simulink model "threee_way"  (R2025b)
settings: Solver=VariableStepAuto  StartTime=0.0  StopTime=0.002  RelTol=1e-3
undefined symbols (not defined in the file or in its folder): dspblkCoreblockFVToolHelper, gcbh
libraries: simulink x4
settings Model: Creator=janek  LastModifiedBy=janek

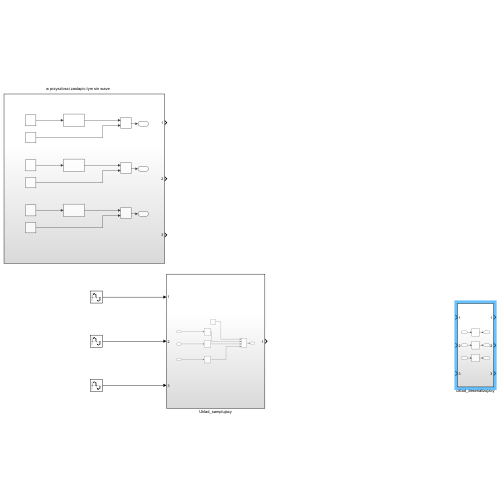
[thumbnail: Simulink's stored preview of the top-level diagram]
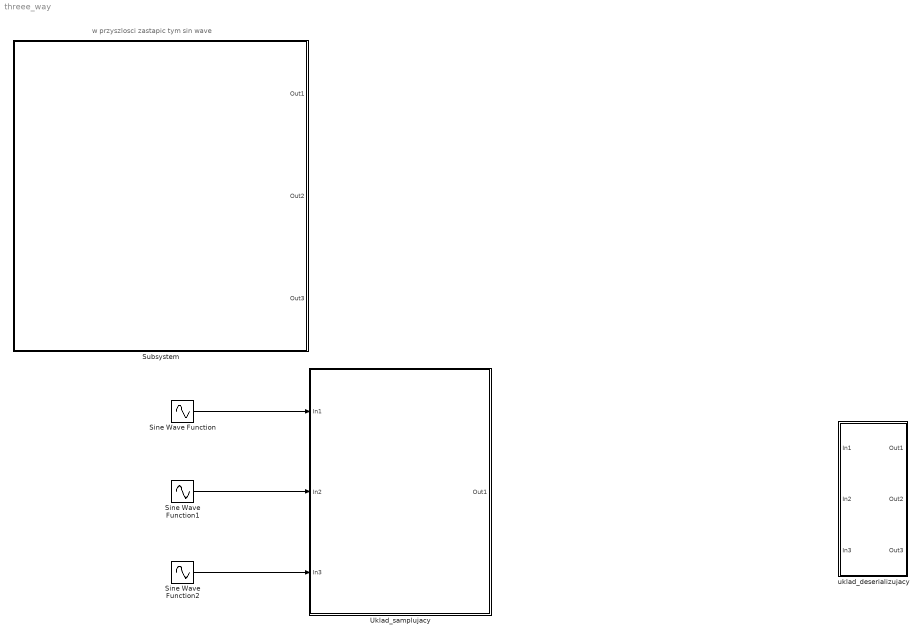
== system threee_way ==
  note: w przyszlosci zastapic tym sin wave
  Sine Wave Function : Sin  Frequency=2*pi*4000  SampleTime=1/27000
  Sine Wave Function1 : Sin  Frequency=2*pi*5000  SampleTime=1/27000
  Sine Wave Function2 : Sin  Frequency=2*pi*3000  SampleTime=1/27000
  Subsystem : Subsystem
  Uklad_samplujacy : Subsystem
  uklad_deserializujacy : Subsystem
  wires:
  Sine Wave Function/1 -> Uklad_samplujacy/1(In1)
  Sine Wave Function1/1 -> Uklad_samplujacy/2(In2)
  Sine Wave Function2/1 -> Uklad_samplujacy/3(In3)

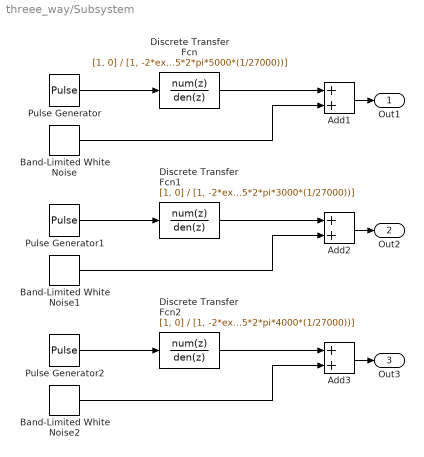
== system threee_way/Subsystem ==
  Add1 : Sum
  Add2 : Sum
  Add3 : Sum
  Band-Limited White Noise : simulink/Sources/Band-Limited White Noise  Cov=[0.000005]  Ts=1/27000  seed=[23341]
  Band-Limited White Noise1 : simulink/Sources/Band-Limited White Noise  Cov=[0.000005]  Ts=1/27000  seed=[23341]
  Band-Limited White Noise2 : simulink/Sources/Band-Limited White Noise  Cov=[0.000005]  Ts=1/27000  seed=[23341]
  Discrete Transfer Fcn : DiscreteTransferFcn  LoadFcn=dspblkCoreblockFVToolHelper(gcbh,'load');  Numerator=[1, 0]  Denominator=[1, -2*exp(-0.05*2*pi*5000*(1/27000))*cos(2*pi*5000*sqrt(1-0.05^2)*(1/27000)), exp(-2*0.05*2*pi*5000*(1/27000))]
      settings: CopyFcn=dspblkCoreblockFVToolHelper(gcbh,'copy');  DeleteFcn=dspblkCoreblockFVToolHelper(gcbh,'close');  ModelCloseFcn=dspblkCoreblockFVToolHelper(gcbh,'close');  PreSaveFcn=dspblkCoreblockFVToolHelper(gcbh,'presave');  PostSaveFcn=dspblkCoreblockFVToolHelper(gcbh,'postsave');  CloseFcn=dspblkCoreblockFVToolHelper(gcbh,'close');
  Discrete Transfer Fcn1 : DiscreteTransferFcn  LoadFcn=dspblkCoreblockFVToolHelper(gcbh,'load');  Numerator=[1, 0]  Denominator=[1, -2*exp(-0.05*2*pi*5000*(1/27000))*cos(2*pi*3000*sqrt(1-0.05^2)*(1/27000)), exp(-2*0.05*2*pi*3000*(1/27000))]
      settings: CopyFcn=dspblkCoreblockFVToolHelper(gcbh,'copy');  DeleteFcn=dspblkCoreblockFVToolHelper(gcbh,'close');  ModelCloseFcn=dspblkCoreblockFVToolHelper(gcbh,'close');  PreSaveFcn=dspblkCoreblockFVToolHelper(gcbh,'presave');  PostSaveFcn=dspblkCoreblockFVToolHelper(gcbh,'postsave');  CloseFcn=dspblkCoreblockFVToolHelper(gcbh,'close');
  Discrete Transfer Fcn2 : DiscreteTransferFcn  LoadFcn=dspblkCoreblockFVToolHelper(gcbh,'load');  Numerator=[1, 0]  Denominator=[1, -2*exp(-0.05*2*pi*5000*(1/27000))*cos(2*pi*4000*sqrt(1-0.05^2)*(1/27000)), exp(-2*0.05*2*pi*4000*(1/27000))]
      settings: CopyFcn=dspblkCoreblockFVToolHelper(gcbh,'copy');  DeleteFcn=dspblkCoreblockFVToolHelper(gcbh,'close');  ModelCloseFcn=dspblkCoreblockFVToolHelper(gcbh,'close');  PreSaveFcn=dspblkCoreblockFVToolHelper(gcbh,'presave');  PostSaveFcn=dspblkCoreblockFVToolHelper(gcbh,'postsave');  CloseFcn=dspblkCoreblockFVToolHelper(gcbh,'close');
  Pulse Generator : DiscretePulseGenerator  PulseType=Time based  Period=1/50  PulseWidth=0.1
  Pulse Generator1 : DiscretePulseGenerator  PulseType=Time based  Period=1/30  PulseWidth=0.1
  Pulse Generator2 : DiscretePulseGenerator  PulseType=Time based  Period=1/40  PulseWidth=0.1
  Out1 : Outport
  Out2 : Outport  Port=2
  Out3 : Outport  Port=3
  wires:
  Discrete Transfer Fcn1/1 -> Add2/1
  Band-Limited White Noise2/1 -> Add3/2
  Band-Limited White Noise1/1 -> Add2/2
  Pulse Generator2/1 -> Discrete Transfer Fcn2/1
  Pulse Generator1/1 -> Discrete Transfer Fcn1/1
  Band-Limited White Noise/1 -> Add1/2
  Pulse Generator/1 -> Discrete Transfer Fcn/1
  Discrete Transfer Fcn/1 -> Add1/1
  Discrete Transfer Fcn2/1 -> Add3/1
  Add1/1 -> Out1/1
  Add2/1 -> Out2/1
  Add3/1 -> Out3/1

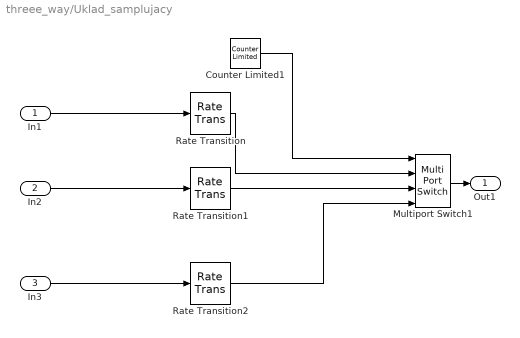
== system threee_way/Uklad_samplujacy ==
  In1 : Inport
  In2 : Inport  Port=2
  In3 : Inport  Port=3
  Counter Limited1 : simulink/Sources/Counter Limited  uplimit=2  tsamp=1/81000
  Multiport Switch1 : MultiPortSwitch  DataPortOrder=Zero-based contiguous  zeroidx=on  SaturateOnIntegerOverflow=off  InputSameDT=off
  Rate Transition : RateTransition  OutPortSampleTime=1/81000
  Rate Transition1 : RateTransition  OutPortSampleTime=1/81000
  Rate Transition2 : RateTransition  OutPortSampleTime=1/81000
  Out1 : Outport
  wires:
  In1/1 -> Rate Transition/1
  Rate Transition2/1 -> Multiport Switch1/4
  Counter Limited1/1 -> Multiport Switch1/1
  Rate Transition1/1 -> Multiport Switch1/3
  In2/1 -> Rate Transition1/1
  Rate Transition/1 -> Multiport Switch1/2
  In3/1 -> Rate Transition2/1
  Multiport Switch1/1 -> Out1/1

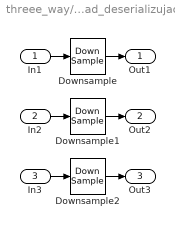
== system threee_way/uklad_deserializujacy ==
  In1 : Inport
  In2 : Inport  Port=2
  In3 : Inport  Port=3
  Downsample : DownSample  N=3  AllowArbitraryFixedInput=on
  Downsample1 : DownSample  N=3  phase=1  AllowArbitraryFixedInput=on
  Downsample2 : DownSample  N=3  phase=2  AllowArbitraryFixedInput=on
  Out1 : Outport
  Out2 : Outport  Port=2
  Out3 : Outport  Port=3
  wires:
  In3/1 -> Downsample2/1
  In1/1 -> Downsample/1
  Downsample/1 -> Out1/1
  In2/1 -> Downsample1/1
  Downsample2/1 -> Out3/1
  Downsample1/1 -> Out2/1
